simulink model "model_obsv_state3disc"  (Simulink 8.7)
settings: Solver=ode45  StartTime=0.0  StopTime=12  MaxStep=1e-3  RelTol=1e-3
values from neighbouring files (symbols this model uses):
  C = [1 0 0 0; 0 0 1 0]    [pendulum_nxt.m]
  J = 0.5*(35.83/2000)*(28/1000)^2    (= 7.02268e-06)    [constants.m]
  K = [-14.8575887588377,-1.51432669500127,-9.99999991426739,-6.51440835206267]    [pendulum_nxt.m]
  L = (80/1000)    (= 0.08)    [constants.m]
  L1 = place(A',C',new_poles)'    [pendulum_nxt.m]
  m = 0.5615    [constants.m]
  N_bar = -inv(Cn*((A-B*K1)\B))    [pendulum_nxt.m]
  r = 0.028    [constants.m]
undefined symbols (not defined in the file or in its folder): A, B, DiscIntNeverNeededParam
undefined symbols (not defined in the file): M
settings Model: Creator=Patrick  LastModifiedBy=WadeJensen
settings DataIOCC: SignalLoggingSaveFormat=ModelDataLogs
settings OptimizationCC: ExpressionDepthLimit=2147483647
settings DebuggingCC: SolverPrmCheckMsg=warning  FcnCallInpInsideContextMsg=EnableAllAsWarning  StateNameClashWarn=warning
settings GRTTargetCC: CombineOutputUpdateFcns=off  GRTInterface=on

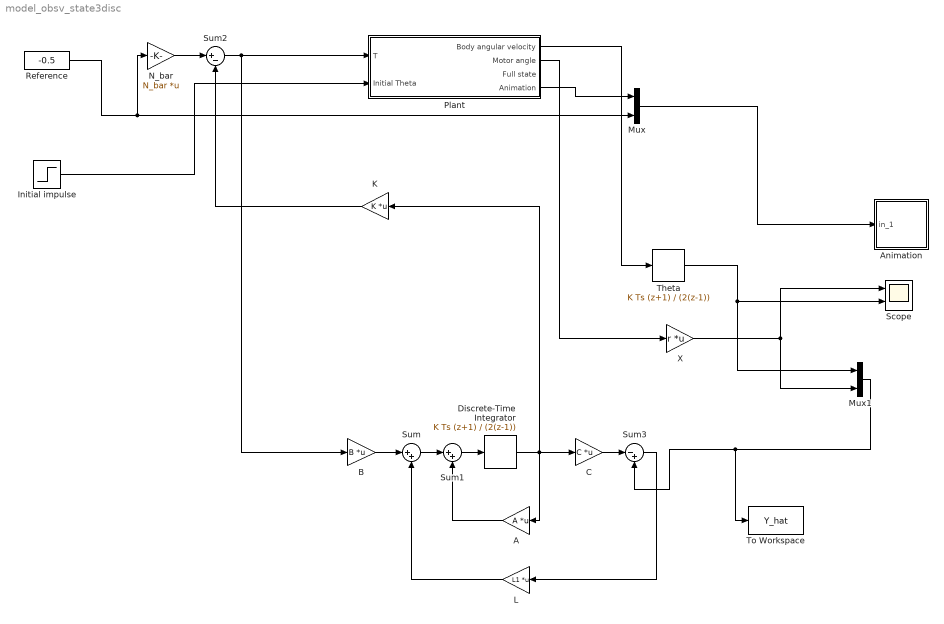
== system model_obsv_state3disc ==
  A : Gain  Gain=A  Multiplication=Matrix(K*u)
  Animation : Subsystem  mask(Pendulum plot){RefBlock=Reference, L=L, r=r, Ts=1e-3}
      mask prompts: RefBlock "DC reference signal block name:"; L "Location of mass"; r "Radius of wheel"; Ts "Simulation time step"
      mask help: Pendulum plot
      mask Help: Pendulum animation function using Handle graphics.
      mask Display: plot([-10 10],[0 0],[-2 -2 2 2],[0 1 1 0],[0 3],[1 5])
  B : Gain  Gain=B  Multiplication=Matrix(K*u)
  C : Gain  Gain=C  Multiplication=Matrix(K*u)
  Discrete-Time Integrator : DiscreteIntegrator  IntegratorMethod=Integration: Trapezoidal  InitialConditionSetting=State (most efficient)  SampleTime=0.00344  ICPrevOutput=DiscIntNeverNeededParam  ICPrevScaledInput=DiscIntNeverNeededParam
  "Initial impulse " : Step  Time=6  After=0  SampleTime=0
  K : Gain  Gain=K  Multiplication=Matrix(K*u)
  L : Gain  Gain=L1  Multiplication=Matrix(K*u)
  Mux : Mux  Inputs=2
  Mux1 : Mux  Inputs=2
  N_bar : Gain  Gain=N_bar  Multiplication=Matrix(K*u)
  Plant : Subsystem  mask{m=m, mw=M, J=J, r=r, L=L, g=9.81, theta0=0.1}
      mask prompts: m "Mass of body"; mw "Mass of wheel"; J "Inertia of wheel"; r "Radius of wheel"; L "Height of body COM"; g "Gravity"; theta0 "Initial angle"
  Reference : Constant  Value=-0.5
  Scope : Scope  NumInputPorts=2
  Sum : Sum  Inputs=|++
  Sum1 : Sum  Inputs=|++
  Sum2 : Sum  Inputs=|+-
  Sum3 : Sum  Inputs=|-+
  "Theta " : DiscreteIntegrator  IntegratorMethod=Integration: Trapezoidal  InitialConditionSetting=State (most efficient)  SampleTime=0.00344  ICPrevOutput=DiscIntNeverNeededParam  ICPrevScaledInput=DiscIntNeverNeededParam
  To Workspace : ToWorkspace  VariableName=Y_hat  SaveFormat=Timeseries  SampleTime=-1
  X : Gain  Gain=r  Multiplication=Matrix(K*u)
  wires:
  Plant/4(Animation) -> Mux/1
  K/1 -> Sum2/2
  A/1 -> Sum1/2
  Sum/1 -> Sum1/1
  B/1 -> Sum/1
  C/1 -> Sum3/1
  Sum3/1 -> L/1
  L/1 -> Sum/2
  Sum2/1 -> B/1, Plant/1(T)
  Plant/2(Motor angle) -> X/1
  X/1 -> Scope/1, Mux1/2
  Mux1/1 -> To Workspace/1, Sum3/2
  N_bar/1 -> Sum2/1
  Reference/1 -> Mux/2, N_bar/1
  "Initial impulse "/1 -> Plant/2(Initial Theta)
  Mux/1 -> Animation/1(in_1)
  Plant/1(Body angular velocity) -> "Theta "/1
  Sum1/1 -> Discrete-Time Integrator/1
  Discrete-Time Integrator/1 -> K/1, A/1, C/1
  "Theta "/1 -> Scope/2, Mux1/1

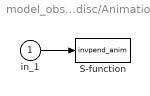
== system model_obsv_state3disc/Animation ==
  in_1 : Inport
  S-function : S-Function  FunctionName=invpend_anim  Parameters=RefBlock,L,r,Ts  SFunctionDeploymentMode=off  EnableBusSupport=off
      settings: DeleteFcn=pendan([],[],[],'DeleteBlock');
  wires:
  in_1/1 -> S-function/1

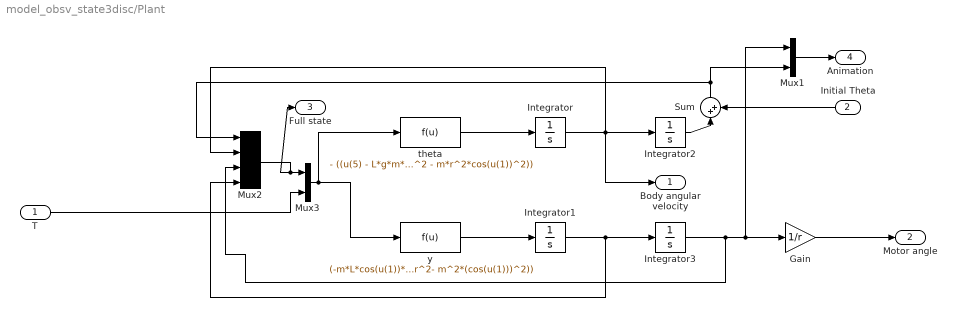
== system model_obsv_state3disc/Plant ==
  T : Inport
  Initial Theta : Inport  Port=2
  Gain : Gain  Gain=1/r
  Integrator{,1..3} (4 alike) : Integrator
  Mux1 : Mux  Inputs=2
  Mux2 : Mux
  Mux3 : Mux  Inputs=2
  Sum : Sum  Inputs=|++
  theta : Fcn  Expr=- ((u(5) - L*g*m*sin(u(1)))*(J + m*r^2 + mw*r^2))/(L^2*m*(J + m*r^2 + mw*r^2 - m*r^2*cos(u(1))^2)) - (r^2*cos(u(1))*(u(5)/r + L*m*u(2)^2*sin(u(1))))/(L*(J + m*r^2 + mw*r^2 - m*r^2*cos(u(1))^2))
  y : Fcn  Expr=(-m*L*cos(u(1))*(m*g*L*sin(u(1)) - u(5)) + m*L^2*(m*L*u(2)^2*sin(u(1))+u(5)/r))/(L^2*(m^2+m*mw+(m*J)/r^2- m^2*(cos(u(1)))^2))
  Body angular velocity : Outport
  Motor angle : Outport  Port=2
  Full state : Outport  Port=3
  Animation : Outport  Port=4
  wires:
  y/1 -> Integrator1/1
  Integrator/1 -> Body angular velocity/1, Integrator2/1, Mux2/2
  Integrator1/1 -> Integrator3/1, Mux2/4
  Integrator3/1 -> Gain/1, Mux1/1, Mux2/3
  T/1 -> Mux3/2
  Gain/1 -> Motor angle/1
  Integrator2/1 -> Sum/1
  Sum/1 -> Mux1/2, Mux2/1
  Initial Theta/1 -> Sum/2
  Mux1/1 -> Animation/1
  Mux2/1 -> Full state/1, Mux3/1
  Mux3/1 -> theta/1, y/1
  theta/1 -> Integrator/1
